simulink model "Prosthesis"  (R2014a)
settings: Solver=ode15s  StartTime=0.0  StopTime=20  MaxStep=.01  RelTol=1e-4  AbsTol=1e-5
InitFcn:
  | RphiKnee0 = 0*pi/180;
  | RphiAnkle0 = 0;
  | prostheticParams
StartFcn:
  | tic;
StopFcn:
  | toc
values from neighbouring files (symbols this model uses):
  ankleBackDriveGain = 0.8    [prostheticParams.m]
  ankleDgain = 0.001    [prostheticParams.m]
  ankleFilterPID = 100    [prostheticParams.m]
  ankleFilterSEA = 100    [prostheticParams.m]
  ankleGearEff = 1.00    (= 1)    [prostheticParams.m]
  ankleGearRatio = 50    [prostheticParams.m]
  ankleIgain = 0.00    (= 0)    [prostheticParams.m]
  ankleInitialAngle = -RphiAnkle0    [prostheticParams.m]
  ankleInputMass = 2329.69    [prostheticParams.m]
  ankleParallelSpringDamping = ankleParallelSpringStiffness/200    (= 0.95)    [prostheticParams.m]
  ankleParallelSpringOffset = 0    [prostheticParams.m]
  ankleParallelSpringStiffness = 190    [prostheticParams.m]
  anklePgain = 0.01    [prostheticParams.m]
  ankleSEADamping = ankleSEAStiffness/100    (= 15)    [prostheticParams.m]
  ankleSEAStiffness = 1500    [prostheticParams.m]
  ankleTendonMass = 36.26    [prostheticParams.m]
  footMassp = 690.10    (= 690.1)    [prostheticParams.m]
  FourBarL1 = 0.080    (= 0.08)    [prostheticParams.m]
  FourBarL3 = 0.0826238    [prostheticParams.m]
  kneeBackDriveGain = 0.8    [prostheticParams.m]
  kneeDgain = 0.001    [prostheticParams.m]
  kneeFilterPID = 100    [prostheticParams.m]
  kneeFilterSEA = 100    [prostheticParams.m]
  kneeGearEff = 1.00    (= 1)    [prostheticParams.m]
  kneeGearRatio = 50    [prostheticParams.m]
  kneeIgain = 0.00    (= 0)    [prostheticParams.m]
  kneeInitialAngle = -RphiKnee0    [prostheticParams.m]
  kneePgain = 0.01    [prostheticParams.m]
  kneeSEADamping = kneeSEAStiffness/100    (= 15)    [prostheticParams.m]
  kneeSEAStiffness = 1500    [prostheticParams.m]
  kneeStatorMass = 1519.39    [prostheticParams.m]
  motorBackEMF = 0.09167    [prostheticParams.m]
  motorInductance = 120e-6    (= 0.00012)    [prostheticParams.m]
  motorMaxCurrent = 4.5/motorTorsionalConst    (= 34.6153846154)    [prostheticParams.m]
  motorMaxVoltage = 48    [prostheticParams.m]
  motorResistance = .055    (= 0.055)    [prostheticParams.m]
  motorRotorInertia = motorRotorMomentOfInertia(3)*gcm2TOkgm2    [prostheticParams.m]
  motorRotorMass = 365.43    [prostheticParams.m]
  motorTorsionalConst = 0.130    (= 0.13)    [prostheticParams.m]
  shankMassp = 2329.69    [prostheticParams.m]
undefined symbols (not defined in the file or in its folder): X, Y, Z
undefined symbols (not defined in the file): ankleIntCoulomb, ankleIntDamping, ankleIntStatic, dryFrictionDamping, dryFrictionStiffness, dryFrictionVelThresh, kneeCJointstop, kneeExtCoulomb, kneeExtDamping, kneeExtStatic, kneeIntCoulomb, kneeIntDamping, kneeIntStatic, kneeWMaxJointstop
libraries: sm_lib x41, nesl_utility x16, simulink x4, NeuroMuscularLibrary x1
(part 2 of 2)

== system Prosthesis/Prosthesis/Knee Motor Rotor ==
  CG : sm_lib/Frames and Transforms/Reference Frame  BlockFunction=simmechanics.library.frames_transforms.reference_frame
  Knee Rotor1 : sm_lib/Body Elements/Solid  InertiaType=Custom  Mass=motorRotorMass  MassUnits=g  CenterOfMass=motorRotorCG  CenterOfMassUnits=mm  MomentsOfInertia=motorRotorMomentOfInertia  MomentsOfInertiaUnits=g*cm^2  ProductsOfInertia=motorRotorProductOfInertia  ProductsOfInertiaUnits=g*cm^2  DensityBased=on  Density=1000  DensityUnits=kg/(m^3)  GraphicType=FromGeometry  MarkerShape=Sphere  MarkerSize=10  MarkerSizeUnits=m  GraphicVisPropType=SimpleVisualProperties  GraphicDiffuseColor=[0.5 0.5 0.5]  GraphicSpecularColor=[0.5 0.5 0.5 1.0]  GraphicAmbientColor=[0.15 0.15 0.15 1.0]  GraphicEmissiveColor=[0.0 0.0 0.0 1.0]  GraphicShininess=75  GraphicOpacity=1.0  GeometryShape=FromFile  RectangleSize=[1 1]  RectangleSizeUnits=m  BrickDimensions=[1 1 1]  BrickDimensionUnits=m  CylinderRadius=1  CylinderRadiusUnits=m  CylinderLength=1  CylinderLengthUnits=m  SphereRadius=1  SphereRadiusUnits=m  EllipsoidRadii=[1 1 1]  EllipsoidRadiiUnits=m  ExtrusionCrossSection=[1 1; -1 1; -1 -1; 1 -1]  ExtrusionCrossSectionUnits=m  ExtrusionLength=1  ExtrusionLengthUnits=m  PolygonNumSides=3  PolygonOuterRadius=1  PolygonOuterRadiusUnits=m  ExtGeomFileType=STL  ExtGeomFileName=motorRotor.STL  ExtGeomFileUnits=mm  RevolutionCrossSection=[1 1; 1 -1; 2 -1; 2 1]  RevolutionCrossSectionUnits=m  RevolutionExtent=Full  RevolutionAngle=180  RevolutionAngleUnits=deg  BlockFunction=simmechanics.library.body_elements.solid
  Rigid Transform : sm_lib/Frames and Transforms/Rigid Transform  TranslationMethod=StandardAxis  TranslationLengthUnit=mm  TranslationStandardAxis=+Z  TranslationStandardOffset=4.5  TranslationCartesianOffset=[0 0 0]  TranslationROffset=0  TranslationROffsetUnits=m  TranslationZOffset=0  TranslationZOffsetUnits=m  TranslationThetaOffset=0  TranslationThetaOffsetUnits=deg  RotationMethod=None  RotationAngleUnits=deg  RotationStandardAxis=+Z  RotationAngle=0  RotationArbitraryAxis=[0 0 1]  FollAlignAxisA=+X  BaseAlignAxisA=+Y  FollAlignAxisB=+Y  BaseAlignAxisB=+Z  BlockFunction=simmechanics.library.frames_transforms.rigid_transform
  ToCG : sm_lib/Frames and Transforms/Rigid Transform  TranslationMethod=Cartesian  TranslationLengthUnit=mm  TranslationStandardAxis=+Z  TranslationStandardOffset=0  TranslationCartesianOffset=motorRotorCG  TranslationROffset=0  TranslationROffsetUnits=m  TranslationZOffset=0  TranslationZOffsetUnits=m  TranslationThetaOffset=0  TranslationThetaOffsetUnits=deg  RotationMethod=None  RotationAngleUnits=deg  RotationStandardAxis=+Z  RotationAngle=0  RotationArbitraryAxis=[0 0 1]  FollAlignAxisA=+X  BaseAlignAxisA=+Y  FollAlignAxisB=+Y  BaseAlignAxisB=+Z  BlockFunction=simmechanics.library.frames_transforms.rigid_transform
  Conn1 : PMIOPort  Port=1  Side=Right
  connections:
  Conn1/RConn1 -- Rigid Transform/LConn1
  Rigid Transform/RConn1 -- Knee Rotor1/RConn1 -- ToCG/LConn1
  CG/RConn1 -- ToCG/RConn1

== system Prosthesis/Prosthesis/Knee SEA Control ==
  Motor Speed : Inport
  Load Acceleration : Inport  Port=2
  Measured Torque : Inport  Port=3
  Desired Torque : Inport  Port=4
  Feed Forward : Subsystem
  PID Controller : simulink/Continuous/PID Controller  Controller=PD  TimeDomain=Continuous-time  SampleTime=.001  IntegratorMethod=Forward Euler  FilterMethod=Forward Euler  Form=Parallel  P=kneePgain  I=kneeIgain  D=kneeDgain  N=kneeFilterPID  InitialConditionSource=internal  InitialConditionForIntegrator=0  InitialConditionForFilter=0  ExternalReset=none  LimitOutput=off  UpperSaturationLimit=inf  LowerSaturationLimit=-inf  LinearizeAsGain=on  AntiWindupMode=none  Kb=1  TrackingMode=off  Kt=1  PParamMin=[]  PParamMax=[]  IParamMin=[]  IParamMax=[]  DParamMin=[]  DParamMax=[]  NParamMin=[]  NParamMax=[]  KbParamMin=[]  KbParamMax=[]  KtParamMin=[]  KtParamMax=[]  POutMin=[]  POutMax=[]  IOutMin=[]  IOutMax=[]  DOutMin=[]  DOutMax=[]  NOutMin=[]  NOutMax=[]  KbOutMin=[]  KbOutMax=[]  KtOutMin=[]  KtOutMax=[]  IntegratorOutMin=[]  IntegratorOutMax=[]  FilterOutMin=[]  FilterOutMax=[]  SumOutMin=[]  SumOutMax=[]  SumI1OutMin=[]  SumI1OutMax=[]  SumI2OutMin=[]  SumI2OutMax=[]  SumI3OutMin=[]  SumI3OutMax=[]  SumDOutMin=[]  SumDOutMax=[]  SaturationOutMin=[]  SaturationOutMax=[]  IntegratorContinuousStateAttributes=''  IntegratorStateMustResolveToSignalObject=off  IntegratorRTWStateStorageClass=Auto  FilterContinuousStateAttributes=''  FilterStateMustResolveToSignalObject=off  FilterRTWStateStorageClass=Auto
  Saturation1 : Saturate  UpperLimit=motorMaxVoltage  LowerLimit=-motorMaxVoltage  ZeroCross=off
  Sum : Sum  Inputs=|+-
  Sum1 : Sum  Inputs=+-|
  Motor Voltage : Outport
  wires:
  PID Controller/1 -> Sum1/2
  Feed Forward/1(Computed Motor Voltage) -> Sum1/1
  Motor Speed/1 -> Feed Forward/1(Motor Speed)
  Sum/1 -> PID Controller/1
  Desired Torque/1 -> Sum/1, Feed Forward/3(Desired Torque)
  Measured Torque/1 -> Sum/2  "Meaasured Torque"
  Load Acceleration/1 -> Feed Forward/2(Load Acceleration)
  Sum1/1 -> Saturation1/1
  Saturation1/1 -> Motor Voltage/1

== system Prosthesis/Prosthesis/Knee Stator ==
  CG : sm_lib/Frames and Transforms/Reference Frame  BlockFunction=simmechanics.library.frames_transforms.reference_frame
  Knee Stator Solid : sm_lib/Body Elements/Solid  InertiaType=Custom  Mass=kneeStatorMass  MassUnits=g  CenterOfMass=kneeStatorCG  CenterOfMassUnits=mm  MomentsOfInertia=kneeStatorMomentOfInertia  MomentsOfInertiaUnits=g*cm^2  ProductsOfInertia=kneeStatorProductOfInertia  ProductsOfInertiaUnits=g*cm^2  DensityBased=off  Density=1000  DensityUnits=kg/(m^3)  GraphicType=FromGeometry  MarkerShape=Sphere  MarkerSize=10  MarkerSizeUnits=m  GraphicVisPropType=SimpleVisualProperties  GraphicDiffuseColor=[0.5 0.5 0.5]  GraphicSpecularColor=[0.5 0.5 0.5 1.0]  GraphicAmbientColor=[0.15 0.15 0.15 1.0]  GraphicEmissiveColor=[0.0 0.0 0.0 1.0]  GraphicShininess=75  GraphicOpacity=1  GeometryShape=FromFile  RectangleSize=[1 1]  RectangleSizeUnits=m  BrickDimensions=[1 1 1]  BrickDimensionUnits=m  CylinderRadius=1  CylinderRadiusUnits=m  CylinderLength=1  CylinderLengthUnits=m  SphereRadius=1  SphereRadiusUnits=m  EllipsoidRadii=[1 1 1]  EllipsoidRadiiUnits=m  ExtrusionCrossSection=[1 1; -1 1; -1 -1; 1 -1]  ExtrusionCrossSectionUnits=m  ExtrusionLength=1  ExtrusionLengthUnits=m  PolygonNumSides=3  PolygonOuterRadius=1  PolygonOuterRadiusUnits=m  ExtGeomFileType=STL  ExtGeomFileName=kneeStator.STL  ExtGeomFileUnits=mm  RevolutionCrossSection=[1 1; 1 -1; 2 -1; 2 1]  RevolutionCrossSectionUnits=m  RevolutionExtent=Full  RevolutionAngle=180  RevolutionAngleUnits=deg  BlockFunction=simmechanics.library.body_elements.solid
  Rigid Transform : sm_lib/Frames and Transforms/Rigid Transform  TranslationMethod=Cartesian  TranslationLengthUnit=mm  TranslationStandardAxis=+Z  TranslationStandardOffset=0  TranslationCartesianOffset=[0, 0, -2]  TranslationROffset=0  TranslationROffsetUnits=m  TranslationZOffset=0  TranslationZOffsetUnits=m  TranslationThetaOffset=0  TranslationThetaOffsetUnits=deg  RotationMethod=None  RotationAngleUnits=deg  RotationStandardAxis=+Z  RotationAngle=0  RotationArbitraryAxis=[0 0 1]  FollAlignAxisA=+X  BaseAlignAxisA=+Y  FollAlignAxisB=+Y  BaseAlignAxisB=+Z  BlockFunction=simmechanics.library.frames_transforms.rigid_transform
  To CG : sm_lib/Frames and Transforms/Rigid Transform  TranslationMethod=Cartesian  TranslationLengthUnit=mm  TranslationStandardAxis=+Z  TranslationStandardOffset=0  TranslationCartesianOffset=kneeStatorCG  TranslationROffset=0  TranslationROffsetUnits=m  TranslationZOffset=0  TranslationZOffsetUnits=m  TranslationThetaOffset=0  TranslationThetaOffsetUnits=deg  RotationMethod=None  RotationAngleUnits=deg  RotationStandardAxis=+Z  RotationAngle=0  RotationArbitraryAxis=[0 0 1]  FollAlignAxisA=+Y  BaseAlignAxisA=+Z  FollAlignAxisB=+X  BaseAlignAxisB=+X  BlockFunction=simmechanics.library.frames_transforms.rigid_transform
  Thigh : PMIOPort  Port=1  Side=Right
  Knee Stator : PMIOPort  Port=2  Side=Left
  connections:
  Rigid Transform/LConn1 -- Thigh/RConn1
  Rigid Transform/RConn1 -- Knee Stator/RConn1 -- Knee Stator Solid/RConn1 -- To CG/LConn1
  CG/RConn1 -- To CG/RConn1

== system Prosthesis/Prosthesis/Shank ==
  CG : sm_lib/Frames and Transforms/Reference Frame  BlockFunction=simmechanics.library.frames_transforms.reference_frame
  Shank : sm_lib/Body Elements/Solid  InertiaType=Custom  Mass=shankMassp  MassUnits=g  CenterOfMass=shankCG  CenterOfMassUnits=mm  MomentsOfInertia=shankMomentOfInertia  MomentsOfInertiaUnits=g*cm^2  ProductsOfInertia=shankProductOfInertia  ProductsOfInertiaUnits=g*cm^2  DensityBased=on  Density=1000  DensityUnits=kg/(m^3)  GraphicType=FromGeometry  MarkerShape=Sphere  MarkerSize=10  MarkerSizeUnits=m  GraphicVisPropType=SimpleVisualProperties  GraphicDiffuseColor=[0.5 0.5 0.5]  GraphicSpecularColor=[0.5 0.5 0.5 1.0]  GraphicAmbientColor=[0.15 0.15 0.15 1.0]  GraphicEmissiveColor=[0.0 0.0 0.0 1.0]  GraphicShininess=75  GraphicOpacity=1.0  GeometryShape=FromFile  RectangleSize=[1 1]  RectangleSizeUnits=m  BrickDimensions=[1 1 1]  BrickDimensionUnits=m  CylinderRadius=1  CylinderRadiusUnits=m  CylinderLength=1  CylinderLengthUnits=m  SphereRadius=1  SphereRadiusUnits=m  EllipsoidRadii=[1 1 1]  EllipsoidRadiiUnits=m  ExtrusionCrossSection=[1 1; -1 1; -1 -1; 1 -1]  ExtrusionCrossSectionUnits=m  ExtrusionLength=1  ExtrusionLengthUnits=m  PolygonNumSides=3  PolygonOuterRadius=1  PolygonOuterRadiusUnits=m  ExtGeomFileType=STL  ExtGeomFileName=shankwKneeSEA.STL  ExtGeomFileUnits=mm  RevolutionCrossSection=[1 1; 1 -1; 2 -1; 2 1]  RevolutionCrossSectionUnits=m  RevolutionExtent=Full  RevolutionAngle=180  RevolutionAngleUnits=deg  BlockFunction=simmechanics.library.body_elements.solid
  To Ankle Stator : sm_lib/Frames and Transforms/Rigid Transform  TranslationMethod=StandardAxis  TranslationLengthUnit=mm  TranslationStandardAxis=-Y  TranslationStandardOffset=124.50  TranslationCartesianOffset=[0 0 0]  TranslationROffset=0  TranslationROffsetUnits=m  TranslationZOffset=0  TranslationZOffsetUnits=m  TranslationThetaOffset=0  TranslationThetaOffsetUnits=deg  RotationMethod=None  RotationAngleUnits=deg  RotationStandardAxis=+Z  RotationAngle=0  RotationArbitraryAxis=[0 0 1]  FollAlignAxisA=+Z  BaseAlignAxisA=+Y  FollAlignAxisB=+Y  BaseAlignAxisB=+Z  BlockFunction=simmechanics.library.frames_transforms.rigid_transform
  To CG : sm_lib/Frames and Transforms/Rigid Transform  TranslationMethod=Cartesian  TranslationLengthUnit=mm  TranslationStandardAxis=-Z  TranslationStandardOffset=1.5  TranslationCartesianOffset=shankCG  TranslationROffset=0  TranslationROffsetUnits=m  TranslationZOffset=0  TranslationZOffsetUnits=m  TranslationThetaOffset=0  TranslationThetaOffsetUnits=deg  RotationMethod=None  RotationAngleUnits=deg  RotationStandardAxis=+Z  RotationAngle=0  RotationArbitraryAxis=[0 0 1]  FollAlignAxisA=+X  BaseAlignAxisA=+Y  FollAlignAxisB=+Y  BaseAlignAxisB=+Z  BlockFunction=simmechanics.library.frames_transforms.rigid_transform
  To Foot : sm_lib/Frames and Transforms/Rigid Transform  TranslationMethod=Cartesian  TranslationLengthUnit=mm  TranslationStandardAxis=-Y  TranslationStandardOffset=445.61  TranslationCartesianOffset=[0, -436.9988, 2]  TranslationROffset=0  TranslationROffsetUnits=m  TranslationZOffset=0  TranslationZOffsetUnits=m  TranslationThetaOffset=0  TranslationThetaOffsetUnits=deg  RotationMethod=None  RotationAngleUnits=deg  RotationStandardAxis=+Z  RotationAngle=0  RotationArbitraryAxis=[0 0 1]  FollAlignAxisA=+X  BaseAlignAxisA=+Y  FollAlignAxisB=+Y  BaseAlignAxisB=+Z  BlockFunction=simmechanics.library.frames_transforms.rigid_transform
  Knee Stator : PMIOPort  Port=1  Side=Right
  Ankle Stator : PMIOPort  Port=2  Side=Left
  Ankle : PMIOPort  Port=3  Side=Left
  connections:
  Shank/RConn1 -- To CG/LConn1 -- To Ankle Stator/LConn1 -- Knee Stator/RConn1 -- To Foot/LConn1
  Ankle Stator/RConn1 -- To Ankle Stator/RConn1
  CG/RConn1 -- To CG/RConn1
  Ankle/RConn1 -- To Foot/RConn1

== system Prosthesis/Prosthesis/Ankle Motor/Friction ==
  Velocity : Inport
  Abs : Abs  ZeroCross=off
  Add : Sum  Inputs=+++
  Divide : Product  Inputs=*/*
  Gain : Gain  Gain=sigma0
  Gain1 : Gain  Gain=sigma1
  Gain2 : Gain  Gain=Fv
  Gain3 : Gain  Gain=-1
  Integrator : Integrator  ZeroCross=off
  Subtract : Sum  Inputs=+-
  g(v) : Fcn  Expr=(Fc + (Fs - Fc)*exp(-(u/v_s)^2))/sigma0
  Friction Force : Outport
  wires:
  Velocity/1 -> Gain2/1, g(v)/1, Abs/1, Subtract/1
  Abs/1 -> Divide/1
  Divide/1 -> Subtract/2
  Subtract/1 -> Integrator/1, Gain1/1  "dz/dt"
  g(v)/1 -> Divide/2
  Integrator/1 -> Divide/3, Gain/1  "z"
  Add/1 -> Gain3/1
  Gain3/1 -> Friction Force/1
  Gain1/1 -> Add/3
  Gain/1 -> Add/2
  Gain2/1 -> Add/1

== system Prosthesis/Prosthesis/Ankle Motor/Motor Dynamics ==
  Voltage : Inport
  Speed : Inport  Port=2
  1/Inductance : Gain  Gain=1/motorInductance
  Add : Sum  Inputs=+--
  Integrator : Integrator
  Resistance : Gain  Gain=motorResistance
  Saturation : Saturate  UpperLimit=motorMaxCurrent  LowerLimit=-motorMaxCurrent  ZeroCross=off
  Torsional Constant : Gain  Gain=motorTorsionalConst
  back EMF : Gain  Gain=motorBackEMF
  Torque : Outport
  wires:
  Voltage/1 -> Add/1
  Torsional Constant/1 -> Torque/1  "Torque"
  Speed/1 -> back EMF/1
  Add/1 -> 1/Inductance/1
  1/Inductance/1 -> Integrator/1  "di/dt"
  back EMF/1 -> Add/3
  Resistance/1 -> Add/2
  Saturation/1 -> Resistance/1, Torsional Constant/1  "Current"
  Integrator/1 -> Saturation/1

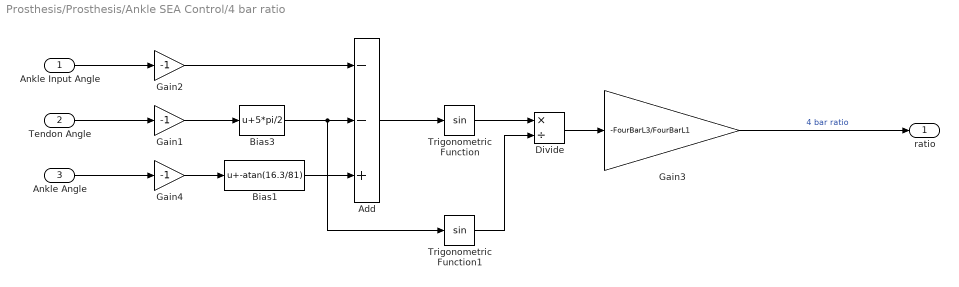
== system Prosthesis/Prosthesis/Ankle SEA Control/4 bar ratio ==
  Ankle Input Angle : Inport
  Tendon Angle : Inport  Port=2
  Ankle Angle : Inport  Port=3
  Add : Sum  Inputs=--+
  Bias1 : Bias  Bias=-atan(16.3/81)
  Bias3 : Bias  Bias=5*pi/2
  Divide : Product  Inputs=*/
  Gain1 : Gain  Gain=-1
  Gain2 : Gain  Gain=-1
  Gain3 : Gain  Gain=-FourBarL3/FourBarL1
  Gain4 : Gain  Gain=-1
  Trigonometric Function : Trigonometry
  Trigonometric Function1 : Trigonometry
  ratio : Outport
  wires:
  Divide/1 -> Gain3/1
  Trigonometric Function1/1 -> Divide/2
  Trigonometric Function/1 -> Divide/1
  Tendon Angle/1 -> Gain1/1
  Add/1 -> Trigonometric Function/1
  Ankle Input Angle/1 -> Gain2/1
  Gain2/1 -> Add/1
  Gain3/1 -> ratio/1  "4 bar ratio"
  Gain4/1 -> Bias1/1
  Ankle Angle/1 -> Gain4/1
  Bias3/1 -> Add/2, Trigonometric Function1/1
  Bias1/1 -> Add/3
  Gain1/1 -> Bias3/1

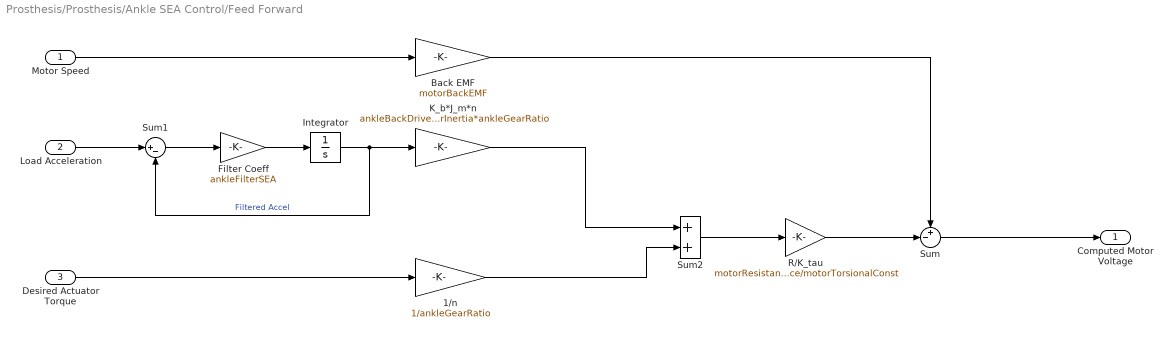
== system Prosthesis/Prosthesis/Ankle SEA Control/Feed Forward ==
  Motor Speed : Inport
  Load Acceleration : Inport  Port=2
  Desired Actuator Torque : Inport  Port=3
  1/n : Gain  Gain=1/ankleGearRatio
  Back EMF : Gain  Gain=motorBackEMF
  Filter Coeff : Gain  Gain=ankleFilterSEA
  Integrator : Integrator
  K_b*J_m*n : Gain  Gain=ankleBackDriveGain*motorRotorInertia*ankleGearRatio
  R/K_tau : Gain  Gain=motorResistance/motorTorsionalConst
  Sum : Sum  Inputs=+-|
  Sum1 : Sum  Inputs=|+-
  Sum2 : Sum
  Computed Motor Voltage : Outport
  wires:
  Sum/1 -> Computed Motor Voltage/1
  K_b*J_m*n/1 -> Sum2/1
  1/n/1 -> Sum2/2
  Desired Actuator Torque/1 -> 1/n/1
  Motor Speed/1 -> Back EMF/1
  R/K_tau/1 -> Sum/2
  Sum2/1 -> R/K_tau/1
  Back EMF/1 -> Sum/1
  Load Acceleration/1 -> Sum1/1
  Integrator/1 -> K_b*J_m*n/1, Sum1/2  "Filtered Accel"
  Sum1/1 -> Filter Coeff/1
  Filter Coeff/1 -> Integrator/1

== system Prosthesis/Prosthesis/Knee Joint/Friction ==
  Velocity : Inport
  Abs : Abs  ZeroCross=off
  Add : Sum  Inputs=+++
  Divide : Product  Inputs=*/*
  Gain : Gain  Gain=sigma0
  Gain1 : Gain  Gain=sigma1
  Gain2 : Gain  Gain=Fv
  Gain3 : Gain  Gain=-1
  Integrator : Integrator  ZeroCross=off
  Subtract : Sum  Inputs=+-
  g(v) : Fcn  Expr=(Fc + (Fs - Fc)*exp(-(u/v_s)^2))/sigma0
  Friction Force : Outport
  wires:
  Velocity/1 -> Gain2/1, g(v)/1, Abs/1, Subtract/1
  Abs/1 -> Divide/1
  Divide/1 -> Subtract/2
  Subtract/1 -> Integrator/1, Gain1/1  "dz/dt"
  g(v)/1 -> Divide/2
  Integrator/1 -> Divide/3, Gain/1  "z"
  Add/1 -> Gain3/1
  Gain3/1 -> Friction Force/1
  Gain1/1 -> Add/3
  Gain/1 -> Add/2
  Gain2/1 -> Add/1

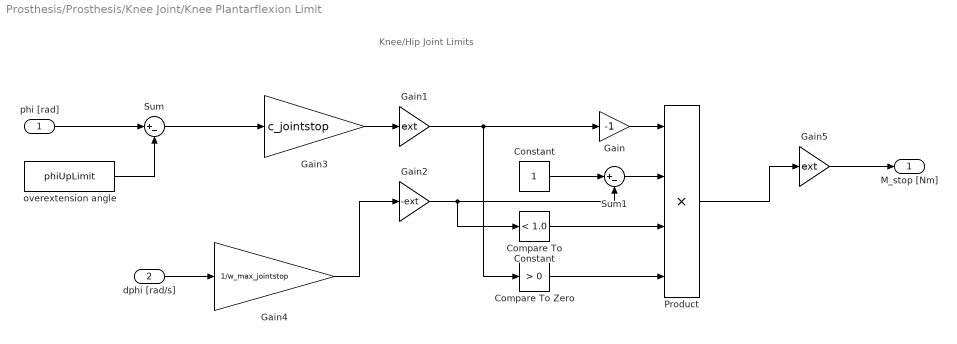
== system Prosthesis/Prosthesis/Knee Joint/Knee Plantarflexion Limit ==
  note: Knee/Hip Joint Limits
  phi [rad] : Inport
  dphi [rad/s] : Inport  Port=2
  Compare To Constant : simulink/Logic and Bit Operations/Compare To Constant  relop=<  const=1.0  OutDataTypeStr=boolean  ZeroCross=off
  Compare To Zero : simulink/Logic and Bit Operations/Compare To Zero  relop=>  OutDataTypeStr=boolean  ZeroCross=off
  Constant : Constant
  Gain : Gain  Gain=-1
  Gain1 : Gain  Gain=ext
  Gain2 : Gain  Gain=-ext
  Gain3 : Gain  Gain=c_jointstop
  Gain4 : Gain  Gain=1/w_max_jointstop
  Gain5 : Gain  Gain=ext
  Product : Product  Inputs=4
  Sum : Sum  Inputs=|+-
  Sum1 : Sum  Inputs=|+-
  overextension angle : Constant  Value=phiUpLimit
  M_stop [Nm] : Outport
  wires:
  Sum/1 -> Gain3/1
  Gain1/1 -> Compare To Zero/1, Gain/1
  Gain3/1 -> Gain1/1
  dphi [rad/s]/1 -> Gain4/1
  overextension angle/1 -> Sum/2
  phi [rad]/1 -> Sum/1
  Gain4/1 -> Gain2/1
  Gain2/1 -> Compare To Constant/1, Sum1/2
  Gain5/1 -> M_stop [Nm]/1
  Constant/1 -> Sum1/1
  Gain/1 -> Product/1
  Sum1/1 -> Product/2
  Compare To Constant/1 -> Product/3
  Compare To Zero/1 -> Product/4
  Product/1 -> Gain5/1

== system Prosthesis/Prosthesis/Knee Motor/Friction ==
  Velocity : Inport
  Abs : Abs  ZeroCross=off
  Add : Sum  Inputs=+++
  Divide : Product  Inputs=*/*
  Gain : Gain  Gain=sigma0
  Gain1 : Gain  Gain=sigma1
  Gain2 : Gain  Gain=Fv
  Gain3 : Gain  Gain=-1
  Integrator : Integrator  ZeroCross=off
  Subtract : Sum  Inputs=+-
  g(v) : Fcn  Expr=(Fc + (Fs - Fc)*exp(-(u/v_s)^2))/sigma0
  Friction Force : Outport
  wires:
  Velocity/1 -> Gain2/1, g(v)/1, Abs/1, Subtract/1
  Abs/1 -> Divide/1
  Divide/1 -> Subtract/2
  Subtract/1 -> Integrator/1, Gain1/1  "dz/dt"
  g(v)/1 -> Divide/2
  Integrator/1 -> Divide/3, Gain/1  "z"
  Add/1 -> Gain3/1
  Gain3/1 -> Friction Force/1
  Gain1/1 -> Add/3
  Gain/1 -> Add/2
  Gain2/1 -> Add/1

== system Prosthesis/Prosthesis/Knee Motor/Motor Dynamics ==
  Voltage : Inport
  Speed : Inport  Port=2
  1/Inductance : Gain  Gain=1/motorInductance
  Add : Sum  Inputs=+--
  Integrator : Integrator
  Resistance : Gain  Gain=motorResistance
  Saturation : Saturate  UpperLimit=motorMaxCurrent  LowerLimit=-motorMaxCurrent  ZeroCross=off
  Torsional Constant : Gain  Gain=motorTorsionalConst
  back EMF : Gain  Gain=motorBackEMF
  Torque : Outport
  wires:
  Voltage/1 -> Add/1
  Torsional Constant/1 -> Torque/1  "Torque"
  Speed/1 -> back EMF/1
  Add/1 -> 1/Inductance/1
  1/Inductance/1 -> Integrator/1  "di/dt"
  back EMF/1 -> Add/3
  Resistance/1 -> Add/2
  Saturation/1 -> Resistance/1, Torsional Constant/1  "Current"
  Integrator/1 -> Saturation/1

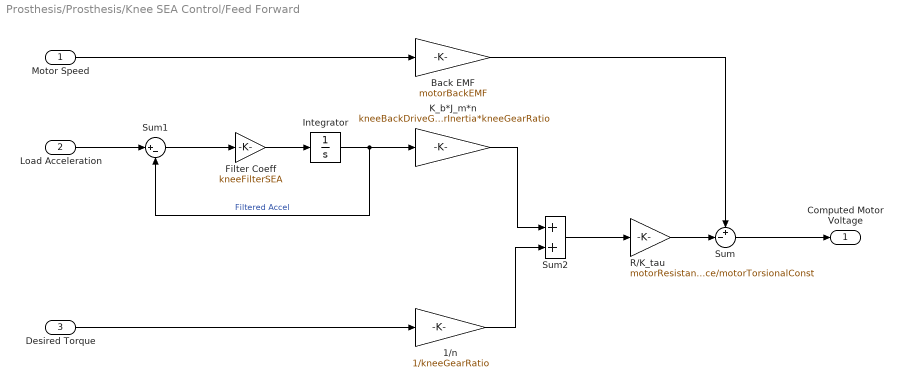
== system Prosthesis/Prosthesis/Knee SEA Control/Feed Forward ==
  Motor Speed : Inport
  Load Acceleration : Inport  Port=2
  Desired Torque : Inport  Port=3
  1/n : Gain  Gain=1/kneeGearRatio
  Back EMF : Gain  Gain=motorBackEMF
  Filter Coeff : Gain  Gain=kneeFilterSEA
  Integrator : Integrator
  K_b*J_m*n : Gain  Gain=kneeBackDriveGain*motorRotorInertia*kneeGearRatio
  R/K_tau : Gain  Gain=motorResistance/motorTorsionalConst
  Sum : Sum  Inputs=+-|
  Sum1 : Sum  Inputs=|+-
  Sum2 : Sum
  Computed Motor Voltage : Outport
  wires:
  Sum/1 -> Computed Motor Voltage/1
  K_b*J_m*n/1 -> Sum2/1
  1/n/1 -> Sum2/2
  Desired Torque/1 -> 1/n/1
  Motor Speed/1 -> Back EMF/1
  R/K_tau/1 -> Sum/2
  Sum2/1 -> R/K_tau/1
  Back EMF/1 -> Sum/1
  Load Acceleration/1 -> Sum1/1
  Integrator/1 -> K_b*J_m*n/1, Sum1/2  "Filtered Accel"
  Sum1/1 -> Filter Coeff/1
  Filter Coeff/1 -> Integrator/1
